simulink model "DAQ"  (R2014a)
settings: Solver=FixedStepDiscrete  StartTime=0.0  StopTime=inf  FixedStep=sample_time  RelTol=1e-3
undefined symbols (not defined in the file): A_lpf_velocity, B1_lpf_velocity, B2_lpf_velocity, BOOM_MAX_ENCODER_TICKS, BOOM_PITCH_CAL_VALUE_RAD, BOOM_PITCH_CAL_VALUE_TICKS, BOOM_PITCH_ENCODER_RAD_PER_TICK, BOOM_ROLL_CAL_VALUE_RAD, BOOM_ROLL_CAL_VALUE_TICKS, BOOM_ROLL_ENCODER_RAD_PER_TICK, BOOM_YAW_ENCODER_RAD_PER_TICK, fcut_smooth, fcut_unwrap, HIP_ABS_ENCODER_RAD_PER_TICK, HIP_ABS_MAX_ENCODER_TICKS, HIP_INC_ENCODER_RAD_PER_TICK, HIP_INC_MAX_ENCODER_TICKS, HIP_MOTOR_CONSTANT, HIP_MTR_GEAR_RATIO, HIP_MTR_MAX_TORQUE, INC_ENC_DIRS, INC_ENC_RAD_PER_TICK, LEFT_HIP_CALIB_POS, LEFT_HIP_CALIB_VAL, LEFT_MOTOR_HIP_DIRECTION, LEG1_LEG_A_CALIB_VAL, LEG1_LEG_A_RAD_PER_CNT, LEG1_LEG_B_CALIB_VAL, LEG1_LEG_B_RAD_PER_CNT, LEG1_MOTOR_A_DIRECTION, LEG1_MOTOR_B_DIRECTION, LEG1_TRAN_A_CALIB_VAL, LEG1_TRAN_A_RAD_PER_CNT, LEG1_TRAN_B_CALIB_VAL, LEG1_TRAN_B_RAD_PER_CNT, LEG2_LEG_A_CALIB_VAL, LEG2_LEG_A_RAD_PER_CNT, LEG2_LEG_B_CALIB_VAL, LEG2_LEG_B_RAD_PER_CNT, LEG2_MOTOR_A_DIRECTION, LEG2_MOTOR_B_DIRECTION, LEG2_TRAN_A_CALIB_VAL, LEG2_TRAN_A_RAD_PER_CNT, LEG2_TRAN_B_CALIB_VAL, LEG2_TRAN_B_RAD_PER_CNT, LEG_A_CALIB_LOC, LEG_B_CALIB_LOC, LEG_MOTOR_CONSTANT, LEG_MTR_GEAR_RATIO, LEG_MTR_MAX_TORQUE, max_encoder_velocity, max_sensor_velocity, MEDULLA_ADC_MAX_VOLTS, MEDULLA_ADC_OFFSET_COUNTS, MEDULLA_TIMER_FREQ, MTR_HIP_MAX_CURRENT, MTR_MAX_COUNT, MTR_MAX_CURRENT, RIGHT_HIP_CALIB_POS, RIGHT_HIP_CALIB_VAL ... (+3)
libraries: xpcethercatlib x174, simulink x18, dspswit3 x1
(part 3 of 3)

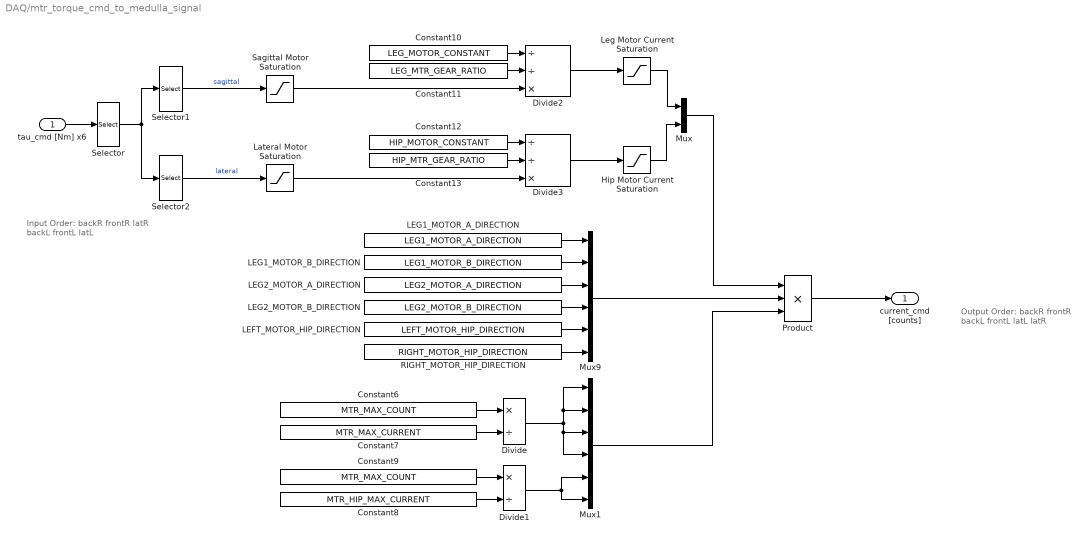
== system DAQ/mtr_torque_cmd_to_medulla_signal ==
  note: Output Order:
      |
      | backR
      | frontR
      | backL
      | frontL
      | latL
      | latR
  note: Input Order:
      |
      | backR
      | frontR
      | latR
      | backL
      | frontL
      | latL
  tau_cmd [Nm] x6 : Inport
  Constant10 : Constant  Value=LEG_MOTOR_CONSTANT
  Constant11 : Constant  Value=LEG_MTR_GEAR_RATIO
  Constant12 : Constant  Value=HIP_MOTOR_CONSTANT
  Constant13 : Constant  Value=HIP_MTR_GEAR_RATIO
  Constant6 : Constant  Value=MTR_MAX_COUNT
  Constant7 : Constant  Value=MTR_MAX_CURRENT
  Constant8 : Constant  Value=MTR_HIP_MAX_CURRENT
  Constant9 : Constant  Value=MTR_MAX_COUNT
  Divide : Product  Inputs=*/
  Divide1 : Product  Inputs=*/
  Divide2 : Product  Inputs=//*
  Divide3 : Product  Inputs=//*
  Hip Motor Current Saturation : Saturate  UpperLimit=10  LowerLimit=-10
      settings: AttributesFormatString=Top: %<UpperLimit>\nBottom: %<LowerLimit>
  LEFT_MOTOR_HIP_DIRECTION : Constant  Value=LEFT_MOTOR_HIP_DIRECTION
  LEG1_MOTOR_A_DIRECTION : Constant  Value=LEG1_MOTOR_A_DIRECTION
  LEG1_MOTOR_B_DIRECTION : Constant  Value=LEG1_MOTOR_B_DIRECTION
  LEG2_MOTOR_A_DIRECTION : Constant  Value=LEG2_MOTOR_A_DIRECTION
  LEG2_MOTOR_B_DIRECTION : Constant  Value=LEG2_MOTOR_B_DIRECTION
  Lateral Motor Saturation : Saturate  UpperLimit=HIP_MTR_MAX_TORQUE  LowerLimit=-HIP_MTR_MAX_TORQUE
      settings: AttributesFormatString=Top: %<UpperLimit>\nBottom: %<LowerLimit>
  Leg Motor Current Saturation : Saturate  UpperLimit=60  LowerLimit=-60
      settings: AttributesFormatString=Top: %<UpperLimit>\nBottom: %<LowerLimit>
  Mux : Mux  Inputs=2
  Mux1 : Mux  Inputs=6
  Mux9 : Mux  Inputs=6
  Product : Product  Inputs=3  RndMeth=Zero
  RIGHT_MOTOR_HIP_DIRECTION : Constant  Value=RIGHT_MOTOR_HIP_DIRECTION
  Sagittal Motor Saturation : Saturate  UpperLimit=LEG_MTR_MAX_TORQUE  LowerLimit=-LEG_MTR_MAX_TORQUE
      settings: AttributesFormatString=Top: %<UpperLimit>\nBottom: %<LowerLimit>
  Selector : Selector  InputPortWidth=6  Indices=[1 2 4 5 6 3]
  Selector1 : Selector  InputPortWidth=6  Indices=[1 2 3 4]
  Selector2 : Selector  InputPortWidth=6  Indices=[5 6]
  current_cmd [counts] : Outport
  wires:
  Lateral Motor Saturation/1 -> Divide3/3
  Sagittal Motor Saturation/1 -> Divide2/3
  Hip Motor Current Saturation/1 -> Mux/2
  Leg Motor Current Saturation/1 -> Mux/1
  Mux/1 -> Product/1
  Divide2/1 -> Leg Motor Current Saturation/1
  Divide3/1 -> Hip Motor Current Saturation/1
  Constant12/1 -> Divide3/1
  Constant13/1 -> Divide3/2
  Constant10/1 -> Divide2/1
  Constant11/1 -> Divide2/2
  Selector2/1 -> Lateral Motor Saturation/1  "lateral"
  Selector1/1 -> Sagittal Motor Saturation/1  "sagittal"
  LEG1_MOTOR_A_DIRECTION/1 -> Mux9/1
  LEG1_MOTOR_B_DIRECTION/1 -> Mux9/2
  LEG2_MOTOR_A_DIRECTION/1 -> Mux9/3
  Mux9/1 -> Product/2
  LEG2_MOTOR_B_DIRECTION/1 -> Mux9/4
  LEFT_MOTOR_HIP_DIRECTION/1 -> Mux9/5
  RIGHT_MOTOR_HIP_DIRECTION/1 -> Mux9/6
  Product/1 -> current_cmd [counts]/1
  Constant6/1 -> Divide/1
  Constant7/1 -> Divide/2
  Divide/1 -> Mux1/4, Mux1/3, Mux1/2, Mux1/1
  Constant9/1 -> Divide1/1
  Constant8/1 -> Divide1/2
  Divide1/1 -> Mux1/6, Mux1/5
  Mux1/1 -> Product/3
  tau_cmd [Nm] x6/1 -> Selector/1
  Selector/1 -> Selector1/1, Selector2/1

== system DAQ/remove_encoder_dropouts ==
  note: predicted value:
      | phi' = phi_(n-1) + dphi
      | = phi_(n-1) + phi_(n-1)-phi_(n-2)
  note: Predict Behavior of Signal
  measured : Inport
  Abs : Abs
  Clock : Clock
  Compare To Zero1 : simulink/Logic and Bit Operations/Compare To Zero  relop=>  OutDataTypeStr=boolean
  Constant : Constant  Value=sensor_start_time+2*sample_time
  Discrete Single Pole Lowpass Filter : DiscreteTransferFcn  Numerator=[(1-exp(-2*pi*fcut_smooth*sample_time)) 0]  Denominator=[1 -exp(-2*pi*fcut_smooth*sample_time)]  SampleTime=sample_time
  Gain2 : Gain  Gain=2
  Sum : Sum  Inputs=|+-
  Sum2 : Sum  Inputs=|+-
  Sum3 : Sum  Inputs=-+|
  Switch : Switch  Criteria=u2 ~= 0  Threshold=max_sensor_velocity*sample_time
      settings: AttributesFormatString=%<Criteria>
  Unit Delay phi_(n-1) : UnitDelay  SampleTime=-1
      settings: AttributesFormatString=initial condition = %<X0>
  Unit Delay phi_(n-2) : UnitDelay  SampleTime=-1
      settings: AttributesFormatString=initial condition = %<X0>
  check_error : Subsystem
  smoothed : Outport
  wires:
  Sum/1 -> Switch/3, Sum3/2  "phi'"
  Gain2/1 -> Sum/1
  Unit Delay phi_(n-1)/1 -> Gain2/1, Unit Delay phi_(n-2)/1
  measured/1 -> Sum3/1, Switch/1  "phi"
  Unit Delay phi_(n-2)/1 -> Sum/2
  Switch/1 -> Discrete Single Pole Lowpass Filter/1, smoothed/1
  Discrete Single Pole Lowpass Filter/1 -> Unit Delay phi_(n-1)/1
  Abs/1 -> check_error/1(error)
  Sum3/1 -> Abs/1  "error"
  check_error/1(acceptable?) -> Switch/2
  Sum2/1 -> Compare To Zero1/1
  Clock/1 -> Sum2/1
  Constant/1 -> Sum2/2
  Compare To Zero1/1 -> check_error/Enable

== system DAQ/unwrap_encoders ==
  Encoder Readings : Inport
  Demux : Demux  Outputs=5
  Mux : Mux  Inputs=6
  Selector : Selector  InputPortWidth=15  Indices=[9 10 11 12 14]
  Selector1 : Selector  InputPortWidth=20  Indices=[1 2 3 4 5 6 7 8 16 17 18 19 13 20 15]
  unwrap_boom_yaw_encoder : Subsystem
  unwrap_lateral_absolute_encoders Left : Subsystem
  unwrap_lateral_absolute_encoders Right : Subsystem
  unwrap_lateral_incremental_encoders Left : Subsystem
  unwrap_lateral_incremental_encoders Right : Subsystem
  Adjusted Encoder Readings : Outport
  wires:
  unwrap_lateral_absolute_encoders Left/1(continuous [ticks]) -> Mux/2
  unwrap_lateral_absolute_encoders Right/1(continuous [ticks]) -> Mux/4
  Demux/3 -> unwrap_lateral_absolute_encoders Right/1(wrapped [ticks])
  Demux/1 -> unwrap_lateral_absolute_encoders Left/1(wrapped [ticks])
  Mux/1 -> Selector1/1
  Selector1/1 -> Adjusted Encoder Readings/1
  unwrap_boom_yaw_encoder/1(continuous [ticks]) -> Mux/6
  unwrap_lateral_incremental_encoders Right/1(continuous [ticks]) -> Mux/5
  unwrap_lateral_incremental_encoders Left/1(continuous [ticks]) -> Mux/3
  Demux/5 -> unwrap_boom_yaw_encoder/1(wrapped [ticks])
  Demux/4 -> unwrap_lateral_incremental_encoders Right/1(wrapped [ticks])
  Demux/2 -> unwrap_lateral_incremental_encoders Left/1(wrapped [ticks])
  Selector/1 -> Demux/1
  Encoder Readings/1 -> Selector/1, Mux/1

== system DAQ/Incremental Encoder Velocity Estimation/Unwrap Encoder ==
  16 bit difference : Inport
  Constant : Constant  Value=2^15
  Constant1 : Constant  Value=2^16
  Constant2 : Constant  Value=2^15
  Sum : Sum  Inputs=|++
  Sum1 : Sum  Inputs=|+-
  modulus : Math  Operator=mod  SaturateOnIntegerOverflow=on
  unwrapped 16 bit difference : Outport
  wires:
  modulus/1 -> Sum1/1
  Constant2/1 -> Sum1/2
  Sum1/1 -> unwrapped 16 bit difference/1
  Constant1/1 -> modulus/2
  Constant/1 -> Sum/2
  16 bit difference/1 -> Sum/1
  Sum/1 -> modulus/1

== system DAQ/calibrate_and_convert_to_rad/calibrate_abs_encoder ==
  encoder_ticks : Inport
  cal_pt_ticks : Inport  Port=2
  cal_pt_rad : Inport  Port=3
  ticks_to_rad_const : Inport  Port=4
  Product : Product  RndMeth=Zero
  Sum : Sum  Inputs=|+-
  Sum1 : Sum  Inputs=|++
  angle [rad] : Outport
  wires:
  Sum/1 -> Product/1  "tick_diff"
  encoder_ticks/1 -> Sum/1  "encoder_ticks"
  Product/1 -> Sum1/1  "rad_diff"
  ticks_to_rad_const/1 -> Product/2  "ticks_to_rad_const"
  cal_pt_ticks/1 -> Sum/2  "calibration_point_ticks"
  Sum1/1 -> angle [rad]/1  "calibrated_angle"
  cal_pt_rad/1 -> Sum1/2  "calibration_point_radians"

== system DAQ/calibrate_and_convert_to_rad/calibration_pt_radians ==
  Constant{1,3,5,7} (4 alike) : Constant  Value=LEG_A_CALIB_LOC
  Constant10 : Constant  Value=LEFT_HIP_CALIB_POS
  Constant11 : Constant  Value=BOOM_ROLL_CAL_VALUE_RAD
  Constant12 : Constant  Value=BOOM_PITCH_CAL_VALUE_RAD
  Constant{2,4,6,8} (4 alike) : Constant  Value=LEG_B_CALIB_LOC
  Constant9 : Constant  Value=RIGHT_HIP_CALIB_POS
  Mux3 : Mux  Inputs=12
  calibration_pt [rad] : Outport
  wires:
  Constant4/1 -> Mux3/4
  Constant8/1 -> Mux3/8
  Constant3/1 -> Mux3/1
  Mux3/1 -> calibration_pt [rad]/1
  Constant11/1 -> Mux3/11
  Constant6/1 -> Mux3/7
  Constant12/1 -> Mux3/12
  Constant9/1 -> Mux3/10
  Constant2/1 -> Mux3/3
  Constant5/1 -> Mux3/6
  Constant1/1 -> Mux3/2
  Constant10/1 -> Mux3/9
  Constant7/1 -> Mux3/5

== system DAQ/calibrate_and_convert_to_rad/calibration_pt_ticks ==
  Constant1 : Constant  Value=LEG2_TRAN_A_CALIB_VAL
  Constant10 : Constant  Value=LEFT_HIP_CALIB_VAL
  Constant11 : Constant  Value=BOOM_ROLL_CAL_VALUE_TICKS
  Constant12 : Constant  Value=BOOM_PITCH_CAL_VALUE_TICKS
  Constant2 : Constant  Value=LEG2_LEG_B_CALIB_VAL
  Constant3 : Constant  Value=LEG2_LEG_A_CALIB_VAL
  Constant4 : Constant  Value=LEG2_TRAN_B_CALIB_VAL
  Constant5 : Constant  Value=LEG1_TRAN_A_CALIB_VAL
  Constant6 : Constant  Value=LEG1_LEG_B_CALIB_VAL
  Constant7 : Constant  Value=LEG1_LEG_A_CALIB_VAL
  Constant8 : Constant  Value=LEG1_TRAN_B_CALIB_VAL
  Constant9 : Constant  Value=RIGHT_HIP_CALIB_VAL
  Mux3 : Mux  Inputs=12
  calibration_pt [ticks] : Outport
  wires:
  Constant3/1 -> Mux3/5
  Constant10/1 -> Mux3/9
  Constant5/1 -> Mux3/2
  Constant1/1 -> Mux3/6
  Constant6/1 -> Mux3/3
  Constant9/1 -> Mux3/10
  Constant12/1 -> Mux3/12
  Constant2/1 -> Mux3/7
  Constant11/1 -> Mux3/11
  Mux3/1 -> calibration_pt [ticks]/1
  Constant7/1 -> Mux3/1
  Constant4/1 -> Mux3/8
  Constant8/1 -> Mux3/4

== system DAQ/calibrate_and_convert_to_rad/ticks_to_radians_constants ==
  Constant1 : Constant  Value=LEG2_TRAN_A_RAD_PER_CNT
  Constant10 : Constant  Value=-HIP_ABS_ENCODER_RAD_PER_TICK
  Constant11 : Constant  Value=BOOM_ROLL_ENCODER_RAD_PER_TICK
  Constant12 : Constant  Value=BOOM_PITCH_ENCODER_RAD_PER_TICK
  Constant2 : Constant  Value=LEG2_LEG_B_RAD_PER_CNT
  Constant3 : Constant  Value=LEG2_LEG_A_RAD_PER_CNT
  Constant4 : Constant  Value=LEG2_TRAN_B_RAD_PER_CNT
  Constant5 : Constant  Value=LEG1_TRAN_A_RAD_PER_CNT
  Constant6 : Constant  Value=LEG1_LEG_B_RAD_PER_CNT
  Constant7 : Constant  Value=LEG1_LEG_A_RAD_PER_CNT
  Constant8 : Constant  Value=LEG1_TRAN_B_RAD_PER_CNT
  Constant9 : Constant  Value=HIP_ABS_ENCODER_RAD_PER_TICK
  Mux3 : Mux  Inputs=12
  ticks_to_rad_constants : Outport
  wires:
  Constant3/1 -> Mux3/5
  Constant9/1 -> Mux3/9
  Constant5/1 -> Mux3/2
  Constant1/1 -> Mux3/6
  Constant6/1 -> Mux3/3
  Constant10/1 -> Mux3/10
  Constant12/1 -> Mux3/12
  Constant2/1 -> Mux3/7
  Constant11/1 -> Mux3/11
  Mux3/1 -> ticks_to_rad_constants/1
  Constant7/1 -> Mux3/1
  Constant4/1 -> Mux3/8
  Constant8/1 -> Mux3/4

== system DAQ/hold_initial_lateral_angles/Initial Lateral Hip Angles [rad] ==
  In : Inport
  Enable : EnablePort  StatesWhenEnabling=reset
  Out : Outport
  wires:
  In/1 -> Out/1

== system DAQ/remove_encoder_dropouts/check_error ==
  error : Inport
  Enable : EnablePort
  Compare To Constant : simulink/Logic and Bit Operations/Compare To Constant  relop=<=  const=max_encoder_velocity*sample_time  OutDataTypeStr=boolean
  acceptable? : Outport  InitialOutput=1
  wires:
  error/1 -> Compare To Constant/1
  Compare To Constant/1 -> acceptable?/1

== system DAQ/unwrap_encoders/unwrap_boom_yaw_encoder ==
  note: Recommended if-then structure for assigning
      | constants. The criterion '~=0' is realized as cpu register
      | shift when compiling.  The resulting code is fast.
  note: Transform Wrapped Angle into Continuous Angle
  note: predicted angle:
      | phi' = phi_(n-1) + dphi
      | = phi_(n-1) + phi_(n-1)-phi_(n-2)
  wrapped [ticks] : Inport
  1/BOOM_MAX_ENCODER_TICKS : Gain  Gain=1/BOOM_MAX_ENCODER_TICKS
  Abs : Abs
  BOOM_MAX_ENCODER_TICKS : Gain  Gain=BOOM_MAX_ENCODER_TICKS
  Compare To Zero : simulink/Logic and Bit Operations/Compare To Zero  relop=>  OutDataTypeStr=uint8
  Discrete Single Pole Lowpass Filter : DiscreteTransferFcn  Numerator=[(1-exp(-2*pi*fcut_unwrap*sample_time)) 0]  Denominator=[1 -exp(-2*pi*fcut_unwrap*sample_time)]  SampleTime=sample_time
  Gain2 : Gain  Gain=2
  Product : Product  RndMeth=Zero
  Rounding Function : Rounding
  Sum : Sum  Inputs=|+-
  Sum1 : Sum  Inputs=|++
  Sum2 : Sum  Inputs=|++
  Sum3 : Sum  Inputs=-+|
  Switch : Switch  Criteria=u2 ~= 0
      settings: AttributesFormatString=%<Criteria>
  Unit Delay phi_(n-1) : UnitDelay  SampleTime=-1
      settings: AttributesFormatString=initial condition = %<X0>
  Unit Delay phi_(n-2) : UnitDelay  SampleTime=-1
      settings: AttributesFormatString=initial condition = %<X0>
  const : Constant  Value=0.5
  no : Constant  Value=-1
  yes : Constant
  continuous [ticks] : Outport
  wires:
  Discrete Single Pole Lowpass Filter/1 -> Unit Delay phi_(n-1)/1
  Compare To Zero/1 -> Switch/2
  Unit Delay phi_(n-2)/1 -> Sum/2
  yes/1 -> Switch/1
  no/1 -> Switch/3
  Switch/1 -> Product/2
  Rounding Function/1 -> BOOM_MAX_ENCODER_TICKS/1
  wrapped [ticks]/1 -> Sum1/1, Sum3/1
  Product/1 -> Sum1/2
  Abs/1 -> 1/BOOM_MAX_ENCODER_TICKS/1
  1/BOOM_MAX_ENCODER_TICKS/1 -> Sum2/1
  const/1 -> Sum2/2
  Sum2/1 -> Rounding Function/1
  Sum1/1 -> continuous [ticks]/1, Discrete Single Pole Lowpass Filter/1
  BOOM_MAX_ENCODER_TICKS/1 -> Product/1
  Unit Delay phi_(n-1)/1 -> Unit Delay phi_(n-2)/1, Gain2/1
  Gain2/1 -> Sum/1
  Sum/1 -> Sum3/2
  Sum3/1 -> Abs/1, Compare To Zero/1  "phi'-phi"

== system DAQ/unwrap_encoders/unwrap_lateral_absolute_encoders Left ==
  note: predicted angle:
      | phi' = phi_(n-1) + dphi
      | = phi_(n-1) + phi_(n-1)-phi_(n-2)
  note: Transform Wrapped Angle into Continuous Angle
  note: Recommended if-then structure for assigning
      | constants. The criterion '~=0' is realized as cpu register
      | shift when compiling.  The resulting code is fast.
  wrapped [ticks] : Inport
  1/HIP_ABS_MAX_ENCODER_TICKS : Gain  Gain=1/HIP_ABS_MAX_ENCODER_TICKS
  Abs : Abs
  Compare To Zero : simulink/Logic and Bit Operations/Compare To Zero  relop=>  OutDataTypeStr=uint8
  Discrete Single Pole Lowpass Filter : DiscreteTransferFcn  Numerator=[(1-exp(-2*pi*fcut_unwrap*sample_time)) 0]  Denominator=[1 -exp(-2*pi*fcut_unwrap*sample_time)]  SampleTime=sample_time
  Gain2 : Gain  Gain=2
  HIP_ABS_MAX_ENCODER_TICKS : Gain  Gain=HIP_ABS_MAX_ENCODER_TICKS
  Product : Product  RndMeth=Zero
  Rounding Function : Rounding
  Sum : Sum  Inputs=|+-
  Sum1 : Sum  Inputs=|++
  Sum2 : Sum  Inputs=|++
  Sum3 : Sum  Inputs=-+|
  Switch : Switch  Criteria=u2 ~= 0
      settings: AttributesFormatString=%<Criteria>
  Unit Delay phi_(n-1) : UnitDelay  SampleTime=-1
      settings: AttributesFormatString=initial condition = %<X0>
  Unit Delay phi_(n-2) : UnitDelay  SampleTime=-1
      settings: AttributesFormatString=initial condition = %<X0>
  const : Constant  Value=0.5
  no : Constant  Value=-1
  yes : Constant
  continuous [ticks] : Outport
  wires:
  Sum3/1 -> Compare To Zero/1, Abs/1  "phi'-phi"
  Sum/1 -> Sum3/2
  Gain2/1 -> Sum/1
  Unit Delay phi_(n-1)/1 -> Gain2/1, Unit Delay phi_(n-2)/1
  HIP_ABS_MAX_ENCODER_TICKS/1 -> Product/1
  Sum1/1 -> continuous [ticks]/1, Discrete Single Pole Lowpass Filter/1
  Sum2/1 -> Rounding Function/1
  const/1 -> Sum2/2
  1/HIP_ABS_MAX_ENCODER_TICKS/1 -> Sum2/1
  Abs/1 -> 1/HIP_ABS_MAX_ENCODER_TICKS/1
  Product/1 -> Sum1/2
  wrapped [ticks]/1 -> Sum3/1, Sum1/1
  Rounding Function/1 -> HIP_ABS_MAX_ENCODER_TICKS/1
  Switch/1 -> Product/2
  no/1 -> Switch/3
  yes/1 -> Switch/1
  Unit Delay phi_(n-2)/1 -> Sum/2
  Compare To Zero/1 -> Switch/2
  Discrete Single Pole Lowpass Filter/1 -> Unit Delay phi_(n-1)/1

== system DAQ/unwrap_encoders/unwrap_lateral_absolute_encoders Right ==
  note: Recommended if-then structure for assigning
      | constants. The criterion '~=0' is realized as cpu register
      | shift when compiling.  The resulting code is fast.
  note: Transform Wrapped Angle into Continuous Angle
  note: predicted angle:
      | phi' = phi_(n-1) + dphi
      | = phi_(n-1) + phi_(n-1)-phi_(n-2)
  wrapped [ticks] : Inport
  1/HIP_ABS_MAX_ENCODER_TICKS : Gain  Gain=1/HIP_ABS_MAX_ENCODER_TICKS
  Abs : Abs
  Compare To Zero : simulink/Logic and Bit Operations/Compare To Zero  relop=>  OutDataTypeStr=uint8
  Discrete Single Pole Lowpass Filter : DiscreteTransferFcn  Numerator=[(1-exp(-2*pi*fcut_unwrap*sample_time)) 0]  Denominator=[1 -exp(-2*pi*fcut_unwrap*sample_time)]  SampleTime=sample_time
  Gain2 : Gain  Gain=2
  HIP_ABS_MAX_ENCODER_TICKS : Gain  Gain=HIP_ABS_MAX_ENCODER_TICKS
  Product : Product  RndMeth=Zero
  Rounding Function : Rounding
  Sum : Sum  Inputs=|+-
  Sum1 : Sum  Inputs=|++
  Sum2 : Sum  Inputs=|++
  Sum3 : Sum  Inputs=-+|
  Switch : Switch  Criteria=u2 ~= 0
      settings: AttributesFormatString=%<Criteria>
  Unit Delay phi_(n-1) : UnitDelay  SampleTime=-1
      settings: AttributesFormatString=initial condition = %<X0>
  Unit Delay phi_(n-2) : UnitDelay  SampleTime=-1
      settings: AttributesFormatString=initial condition = %<X0>
  const : Constant  Value=0.5
  no : Constant  Value=-1
  yes : Constant
  continuous [ticks] : Outport
  wires:
  Discrete Single Pole Lowpass Filter/1 -> Unit Delay phi_(n-1)/1
  Compare To Zero/1 -> Switch/2
  Unit Delay phi_(n-2)/1 -> Sum/2
  yes/1 -> Switch/1
  no/1 -> Switch/3
  Switch/1 -> Product/2
  Rounding Function/1 -> HIP_ABS_MAX_ENCODER_TICKS/1
  wrapped [ticks]/1 -> Sum1/1, Sum3/1
  Product/1 -> Sum1/2
  Abs/1 -> 1/HIP_ABS_MAX_ENCODER_TICKS/1
  1/HIP_ABS_MAX_ENCODER_TICKS/1 -> Sum2/1
  const/1 -> Sum2/2
  Sum2/1 -> Rounding Function/1
  Sum1/1 -> Discrete Single Pole Lowpass Filter/1, continuous [ticks]/1
  HIP_ABS_MAX_ENCODER_TICKS/1 -> Product/1
  Unit Delay phi_(n-1)/1 -> Unit Delay phi_(n-2)/1, Gain2/1
  Gain2/1 -> Sum/1
  Sum/1 -> Sum3/2
  Sum3/1 -> Abs/1, Compare To Zero/1  "phi'-phi"

== system DAQ/unwrap_encoders/unwrap_lateral_incremental_encoders Left ==
  note: Recommended if-then structure for assigning
      | constants. The criterion '~=0' is realized as cpu register
      | shift when compiling.  The resulting code is fast.
  note: Transform Wrapped Angle into Continuous Angle
  note: predicted angle:
      | phi' = phi_(n-1) + dphi
      | = phi_(n-1) + phi_(n-1)-phi_(n-2)
  wrapped [ticks] : Inport
  1/HIP_INC_MAX_ENCODER_TICKS : Gain  Gain=1/HIP_INC_MAX_ENCODER_TICKS
  Abs : Abs
  Compare To Zero : simulink/Logic and Bit Operations/Compare To Zero  relop=>  OutDataTypeStr=uint8
  Discrete Single Pole Lowpass Filter : DiscreteTransferFcn  Numerator=[(1-exp(-2*pi*fcut_unwrap*sample_time)) 0]  Denominator=[1 -exp(-2*pi*fcut_unwrap*sample_time)]  SampleTime=sample_time
  Gain2 : Gain  Gain=2
  HIP_INC_MAX_ENCODER_TICKS : Gain  Gain=HIP_INC_MAX_ENCODER_TICKS
  Product : Product  RndMeth=Zero
  Rounding Function : Rounding
  Sum : Sum  Inputs=|+-
  Sum1 : Sum  Inputs=|++
  Sum2 : Sum  Inputs=|++
  Sum3 : Sum  Inputs=-+|
  Switch : Switch  Criteria=u2 ~= 0
      settings: AttributesFormatString=%<Criteria>
  Unit Delay phi_(n-1) : UnitDelay  SampleTime=-1
      settings: AttributesFormatString=initial condition = %<X0>
  Unit Delay phi_(n-2) : UnitDelay  SampleTime=-1
      settings: AttributesFormatString=initial condition = %<X0>
  const : Constant  Value=0.5
  no : Constant  Value=-1
  yes : Constant
  continuous [ticks] : Outport
  wires:
  Discrete Single Pole Lowpass Filter/1 -> Unit Delay phi_(n-1)/1
  Compare To Zero/1 -> Switch/2
  Unit Delay phi_(n-2)/1 -> Sum/2
  yes/1 -> Switch/1
  no/1 -> Switch/3
  Switch/1 -> Product/2
  Rounding Function/1 -> HIP_INC_MAX_ENCODER_TICKS/1
  wrapped [ticks]/1 -> Sum1/1, Sum3/1
  Product/1 -> Sum1/2
  Abs/1 -> 1/HIP_INC_MAX_ENCODER_TICKS/1
  1/HIP_INC_MAX_ENCODER_TICKS/1 -> Sum2/1
  const/1 -> Sum2/2
  Sum2/1 -> Rounding Function/1
  Sum1/1 -> Discrete Single Pole Lowpass Filter/1, continuous [ticks]/1
  HIP_INC_MAX_ENCODER_TICKS/1 -> Product/1
  Unit Delay phi_(n-1)/1 -> Unit Delay phi_(n-2)/1, Gain2/1
  Gain2/1 -> Sum/1
  Sum/1 -> Sum3/2
  Sum3/1 -> Abs/1, Compare To Zero/1  "phi'-phi"

== system DAQ/unwrap_encoders/unwrap_lateral_incremental_encoders Right ==
  note: predicted angle:
      | phi' = phi_(n-1) + dphi
      | = phi_(n-1) + phi_(n-1)-phi_(n-2)
  note: Transform Wrapped Angle into Continuous Angle
  note: Recommended if-then structure for assigning
      | constants. The criterion '~=0' is realized as cpu register
      | shift when compiling.  The resulting code is fast.
  wrapped [ticks] : Inport
  1/HIP_INC_MAX_ENCODER_TICKS : Gain  Gain=1/HIP_INC_MAX_ENCODER_TICKS
  Abs : Abs
  Compare To Zero : simulink/Logic and Bit Operations/Compare To Zero  relop=>  OutDataTypeStr=uint8
  Discrete Single Pole Lowpass Filter : DiscreteTransferFcn  Numerator=[(1-exp(-2*pi*fcut_unwrap*sample_time)) 0]  Denominator=[1 -exp(-2*pi*fcut_unwrap*sample_time)]  SampleTime=sample_time
  Gain2 : Gain  Gain=2
  HIP_INC_MAX_ENCODER_TICKS : Gain  Gain=HIP_INC_MAX_ENCODER_TICKS
  Product : Product  RndMeth=Zero
  Rounding Function : Rounding
  Sum : Sum  Inputs=|+-
  Sum1 : Sum  Inputs=|++
  Sum2 : Sum  Inputs=|++
  Sum3 : Sum  Inputs=-+|
  Switch : Switch  Criteria=u2 ~= 0
      settings: AttributesFormatString=%<Criteria>
  Unit Delay phi_(n-1) : UnitDelay  SampleTime=-1
      settings: AttributesFormatString=initial condition = %<X0>
  Unit Delay phi_(n-2) : UnitDelay  SampleTime=-1
      settings: AttributesFormatString=initial condition = %<X0>
  const : Constant  Value=0.5
  no : Constant  Value=-1
  yes : Constant
  continuous [ticks] : Outport
  wires:
  Sum3/1 -> Compare To Zero/1, Abs/1  "phi'-phi"
  Sum/1 -> Sum3/2
  Gain2/1 -> Sum/1
  Unit Delay phi_(n-1)/1 -> Gain2/1, Unit Delay phi_(n-2)/1
  HIP_INC_MAX_ENCODER_TICKS/1 -> Product/1
  Sum1/1 -> continuous [ticks]/1, Discrete Single Pole Lowpass Filter/1
  Sum2/1 -> Rounding Function/1
  const/1 -> Sum2/2
  1/HIP_INC_MAX_ENCODER_TICKS/1 -> Sum2/1
  Abs/1 -> 1/HIP_INC_MAX_ENCODER_TICKS/1
  Product/1 -> Sum1/2
  wrapped [ticks]/1 -> Sum3/1, Sum1/1
  Rounding Function/1 -> HIP_INC_MAX_ENCODER_TICKS/1
  Switch/1 -> Product/2
  no/1 -> Switch/3
  yes/1 -> Switch/1
  Unit Delay phi_(n-2)/1 -> Sum/2
  Compare To Zero/1 -> Switch/2
  Discrete Single Pole Lowpass Filter/1 -> Unit Delay phi_(n-1)/1

== matlab function DAQ/logic_voltage_volts ==
  data: u input; volt output; MEDULLA_ADC_OFFSET_COUNTS parameter; MEDULLA_ADC_MAX_VOLTS parameter
function volt = fcn(u, MEDULLA_ADC_OFFSET_COUNTS, MEDULLA_ADC_MAX_VOLTS)
% Taken from Medulla.cpp in the ATRIAS medulla drivers
% at code.google.com/p/atrias
adcReadingVolts = (u - MEDULLA_ADC_OFFSET_COUNTS) * MEDULLA_ADC_MAX_VOLTS/4095;
volt            = 6 * adcReadingVolts;

== matlab function DAQ/medulla_errors ==
  data: u input; errors output
function errors = fcn(u)
% right back, right front, left back, left front, left lateral, right lateral, imu, boom
errors = reshape(bsxfun(@bitand,u,2.^[0 1 2 3 4 5 6 7]),[],1);

== matlab function DAQ/motor_temperatures ==
  data: u input; temp output
function temp = fcn(u)
adc_values = ((u - 172.0) * (2.70/(4095.0)));
temp = ((1.0./( (1.0/298.15) + (1.0/3988.0)*log(4700.0./((3.26./adc_values) - 1.0)/10000))) - 273.15);

== matlab function DAQ/motor_voltage_volts ==
  data: u input; volt output
function volt = fcn(u)
volt = (u - 1300.0) * 60.2 / (3600.0 - 1300.0);
